simulink model "att_control_OneModule_V6"  (R2022a)
settings: Solver=ode15s  StartTime=0.0  StopTime=10  FixedStep=0.001  RelTol=1e-3
values from neighbouring files (symbols this model uses):
  act_lo = 0    [rotors_prg.m]
  act_up = 1000    [rotors_prg.m]
  des_alt = 1    [rotors_prg.m]
  des_p = 0    [rotors_prg.m]
  des_r = 0    [rotors_prg.m]
  des_y = 0    [rotors_prg.m]
  dragCoeffMov = 0    [rotors_prg.m]
  g = 9.81    [rotors_prg.m]
  KDx = 0.003*1    (= 0.003)    [rotors_prg.m]
  KDy = 0.003*1    (= 0.003)    [rotors_prg.m]
  KDz = 0.003*1    (= 0.003)    [rotors_prg.m]
  KIx = 0.2*1    (= 0.2)    [rotors_prg.m]
  KIy = 0.2*1    (= 0.2)    [rotors_prg.m]
  KIz = 0.2*1    (= 0.2)    [rotors_prg.m]
  KP1x = 6.5    [rotors_prg.m]
  KP1y = 6.5    [rotors_prg.m]
  KP1z = 2.8    [rotors_prg.m]
  KP2x = 0.15^1    (= 0.15)    [rotors_prg.m]
  KP2y = 0.15^1    (= 0.15)    [rotors_prg.m]
  KP2z = 0.15^1    (= 0.15)    [rotors_prg.m]
  mass = 16*mass1    (= 14.24)    [rotors_prg.m]
  Mv = inv(M)    [rotors_prg.m]
  rotorDir = rotorDirX    [rotors_prg.m]
  rotorPositions = rotorPositions16    [rotors_prg.m]
  rotorThrustMax = 5.3    [rotors_prg.m]
  rotorTimeConst = 0.005    [rotors_prg.m]
  rotorTorqueMax = 0.078    [rotors_prg.m]
  windVel = [0;0;0]    [rotors_prg.m]
undefined symbols (not defined in the file or in its folder): init
libraries: slpidlib x10, sharedtransform x3, simulink x2, aerolibutil x2, shared6dof x1, sharedutil x1
(part 1 of 2)
settings Model: Creator=MohShahab  LastModifiedBy=MohShahab
settings SolverCC: ZeroCrossAlgorithm=Adaptive
settings DebuggingCC: MaskedZcDiagnostic=none  IgnoredZcDiagnostic=none
settings SFSimCC: SimTargetLang=C++

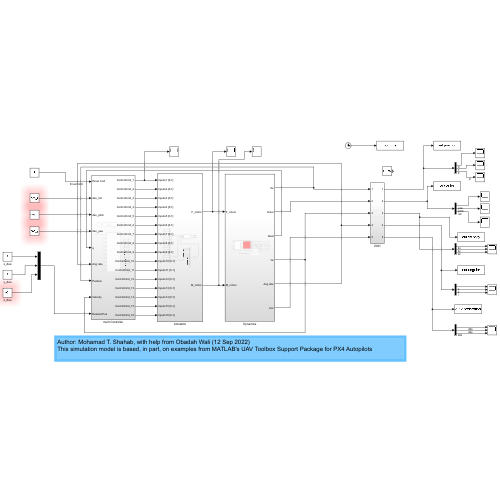
[thumbnail: Simulink's stored preview of the top-level diagram]
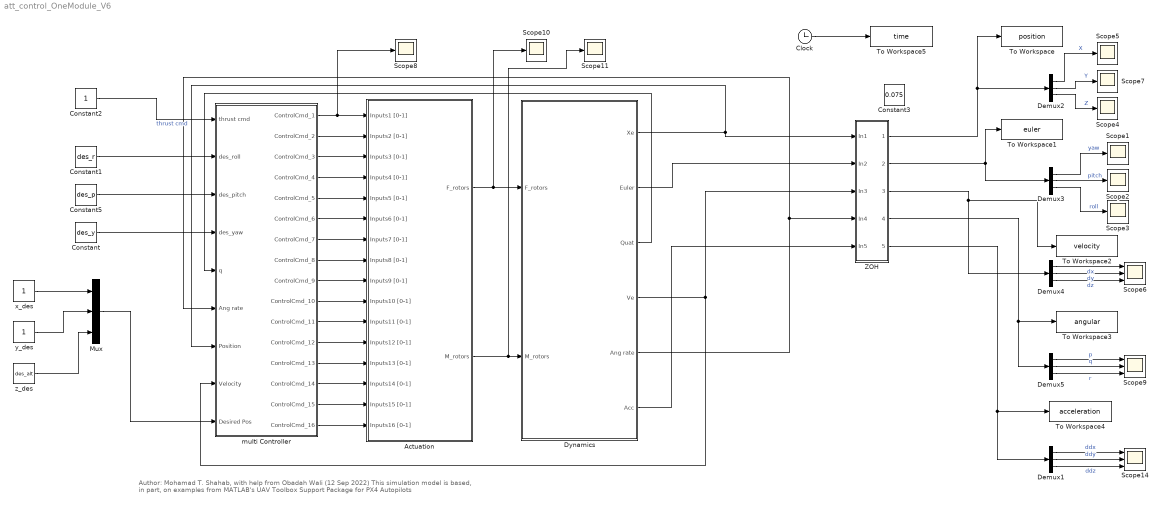
== system att_control_OneModule_V6 ==
  note: Author: Mohamad T. Shahab, with help from Obadah Wali (12 Sep 2022)
      | This simulation model is based, in part, on examples from MATLAB's UAV Toolbox Support Package for PX4 Autopilots
  Actuation : Subsystem
  Clock : Clock
  Constant : Constant  Value=des_y
  Constant1 : Constant  Value=des_r
  Constant2 : Constant
  Constant3 : Constant  Value=0.075
  Constant5 : Constant  Value=des_p
  Demux{1..5} (5 alike) : Demux  Outputs=3
  Dynamics : Subsystem
  Mux : Mux  Inputs=3
  Scope{1..5,7..8,10..11} (9 alike) : Scope
  Scope14 : Scope  NumInputPorts=3
  Scope6 : Scope  NumInputPorts=3
  Scope9 : Scope  NumInputPorts=3
  To Workspace : ToWorkspace  VariableName=position  SaveFormat=Timeseries  SampleTime=-1
  To Workspace1 : ToWorkspace  VariableName=euler  SaveFormat=Timeseries  SampleTime=-1
  To Workspace2 : ToWorkspace  VariableName=velocity  SaveFormat=Timeseries  SampleTime=-1
  To Workspace3 : ToWorkspace  VariableName=angular  SaveFormat=Timeseries  SampleTime=-1
  To Workspace4 : ToWorkspace  VariableName=acceleration  SaveFormat=Timeseries  SampleTime=-1
  To Workspace5 : ToWorkspace  VariableName=time  SaveFormat=Timeseries  SampleTime=-1
  ZOH : Subsystem
  multi Controller : Subsystem
  x_des : Constant
  y_des : Constant
  z_des : Constant  Value=des_alt
  wires:
  Demux5/3 -> Scope9/3  "r"
  Demux4/3 -> Scope6/3  "dz"
  Demux5/2 -> Scope9/2  "q"
  Demux4/1 -> Scope6/1  "dx"
  Demux5/1 -> Scope9/1  "p"
  Demux1/2 -> Scope14/2  "ddy"
  Demux1/1 -> Scope14/1  "ddx"
  Demux2/3 -> Scope4/1  "Z"
  Demux1/3 -> Scope14/3  "ddz"
  Demux4/2 -> Scope6/2  "dy"
  Dynamics/5(Ang rate) -> ZOH/4(In4), multi Controller/6(Ang rate)
  Constant2/1 -> multi Controller/1(thrust cmd)  "thrust cmd"
  Constant1/1 -> multi Controller/2(des_roll)
  Dynamics/3(Quat) -> multi Controller/5(q)
  Constant/1 -> multi Controller/4(des_yaw)
  Constant5/1 -> multi Controller/3(des_pitch)
  Dynamics/1(Xe) -> ZOH/1(In1), multi Controller/7(Position)
  Dynamics/2(Euler) -> ZOH/2(In2)
  Dynamics/4(Ve) -> multi Controller/8(Velocity), ZOH/3(In3)
  Dynamics/6(Acc) -> ZOH/5(In5)
  ZOH/1(Out1) -> Demux2/1, To Workspace/1
  ZOH/3(Out3) -> Demux4/1, To Workspace2/1
  ZOH/4(Out4) -> To Workspace3/1, Demux5/1
  ZOH/5(Out5) -> To Workspace4/1, Demux1/1
  Mux/1 -> multi Controller/9(Desired Pos)
  x_des/1 -> Mux/1
  y_des/1 -> Mux/2
  z_des/1 -> Mux/3
  Demux3/1 -> Scope1/1  "yaw"
  ZOH/2(Out2) -> To Workspace1/1, Demux3/1
  Demux3/2 -> Scope2/1  "pitch"
  multi Controller/1(ControlCmd_1) -> Scope8/1, Actuation/1(Inputs1 [0-1])
  Actuation/1(F_rotors) -> Scope10/1, Dynamics/1(F_rotors)
  Actuation/2(M_rotors) -> Scope11/1, Dynamics/2(M_rotors)
  multi Controller/2(ControlCmd_2) -> Actuation/2(Inputs2 [0-1])
  multi Controller/3(ControlCmd_3) -> Actuation/3(Inputs3 [0-1])
  multi Controller/4(ControlCmd_4) -> Actuation/4(Inputs4 [0-1])
  multi Controller/5(ControlCmd_5) -> Actuation/5(Inputs5 [0-1])
  multi Controller/6(ControlCmd_6) -> Actuation/6(Inputs6 [0-1])
  multi Controller/7(ControlCmd_7) -> Actuation/7(Inputs7 [0-1])
  multi Controller/8(ControlCmd_8) -> Actuation/8(Inputs8 [0-1])
  multi Controller/9(ControlCmd_9) -> Actuation/9(Inputs9 [0-1])
  multi Controller/10(ControlCmd_10) -> Actuation/10(Inputs10 [0-1])
  multi Controller/11(ControlCmd_11) -> Actuation/11(Inputs11 [0-1])
  multi Controller/12(ControlCmd_12) -> Actuation/12(Inputs12 [0-1])
  multi Controller/13(ControlCmd_13) -> Actuation/13(Inputs13 [0-1])
  multi Controller/14(ControlCmd_14) -> Actuation/14(Inputs14 [0-1])
  multi Controller/15(ControlCmd_15) -> Actuation/15(Inputs15 [0-1])
  multi Controller/16(ControlCmd_16) -> Actuation/16(Inputs16 [0-1])
  Demux2/1 -> Scope5/1  "X"
  Demux2/2 -> Scope7/1  "Y"
  Clock/1 -> To Workspace5/1
  Demux3/3 -> Scope3/1  "roll"

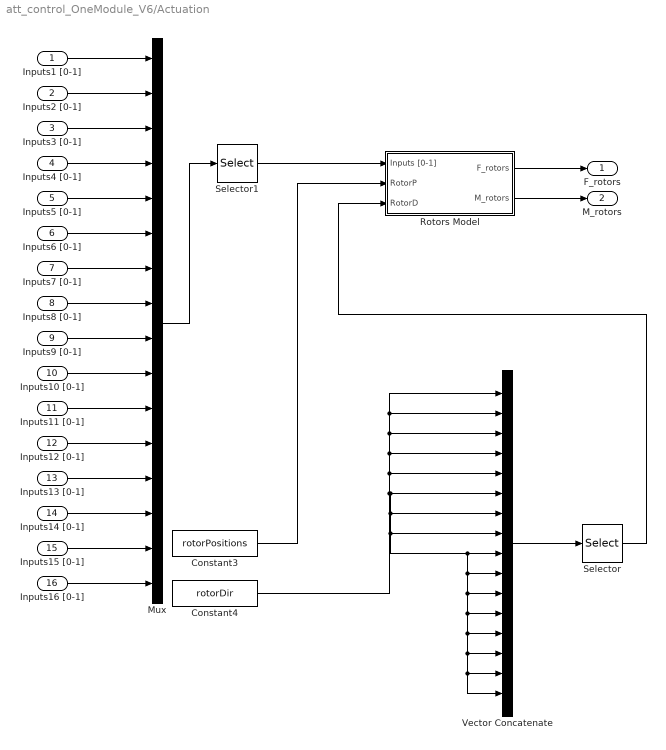
== system att_control_OneModule_V6/Actuation ==
  Inputs1 [0-1] : Inport
  Inputs2 [0-1] : Inport  Port=2
  Inputs3 [0-1] : Inport  Port=3
  Inputs4 [0-1] : Inport  Port=4
  Inputs5 [0-1] : Inport  Port=5
  Inputs6 [0-1] : Inport  Port=6
  Inputs7 [0-1] : Inport  Port=7
  Inputs8 [0-1] : Inport  Port=8
  Inputs9 [0-1] : Inport  Port=9
  Inputs10 [0-1] : Inport  Port=10
  Inputs11 [0-1] : Inport  Port=11
  Inputs12 [0-1] : Inport  Port=12
  Inputs13 [0-1] : Inport  Port=13
  Inputs14 [0-1] : Inport  Port=14
  Inputs15 [0-1] : Inport  Port=15
  Inputs16 [0-1] : Inport  Port=16
  Constant3 : Constant  Value=rotorPositions
  Constant4 : Constant  Value=rotorDir
  Mux : Mux  Inputs=16
  Rotors Model : Subsystem
  Selector : Selector  InputPortWidth=64  IndexOptions=Starting index (dialog)  Indices=1  OutputSizes=NumRotors
  Selector1 : Selector  InputPortWidth=64  IndexOptions=Starting index (dialog)  Indices=1  OutputSizes=NumRotors
  Vector Concatenate : Concatenate  NumInputs=16
  F_rotors : Outport
  M_rotors : Outport  Port=2
  wires:
  Rotors Model/2(M_rotors) -> M_rotors/1
  Rotors Model/1(F_rotors) -> F_rotors/1
  Inputs3 [0-1]/1 -> Mux/3
  Inputs4 [0-1]/1 -> Mux/4
  Constant3/1 -> Rotors Model/2(RotorP)
  Inputs7 [0-1]/1 -> Mux/7
  Inputs8 [0-1]/1 -> Mux/8
  Inputs6 [0-1]/1 -> Mux/6
  Inputs5 [0-1]/1 -> Mux/5
  Inputs11 [0-1]/1 -> Mux/11
  Inputs12 [0-1]/1 -> Mux/12
  Inputs10 [0-1]/1 -> Mux/10
  Inputs9 [0-1]/1 -> Mux/9
  Inputs15 [0-1]/1 -> Mux/15
  Inputs16 [0-1]/1 -> Mux/16
  Inputs14 [0-1]/1 -> Mux/14
  Inputs13 [0-1]/1 -> Mux/13
  Constant4/1 -> Vector Concatenate/2, Vector Concatenate/1, Vector Concatenate/3, Vector Concatenate/4, Vector Concatenate/5, Vector Concatenate/16, Vector Concatenate/15, Vector Concatenate/14, Vector Concatenate/13, Vector Concatenate/12, Vector Concatenate/11, Vector Concatenate/10, Vector Concatenate/9, Vector Concatenate/8, Vector Concatenate/7, Vector Concatenate/6
  Vector Concatenate/1 -> Selector/1
  Selector/1 -> Rotors Model/3(RotorD)
  Mux/1 -> Selector1/1
  Selector1/1 -> Rotors Model/1(Inputs [0-1])
  Inputs2 [0-1]/1 -> Mux/2
  Inputs1 [0-1]/1 -> Mux/1

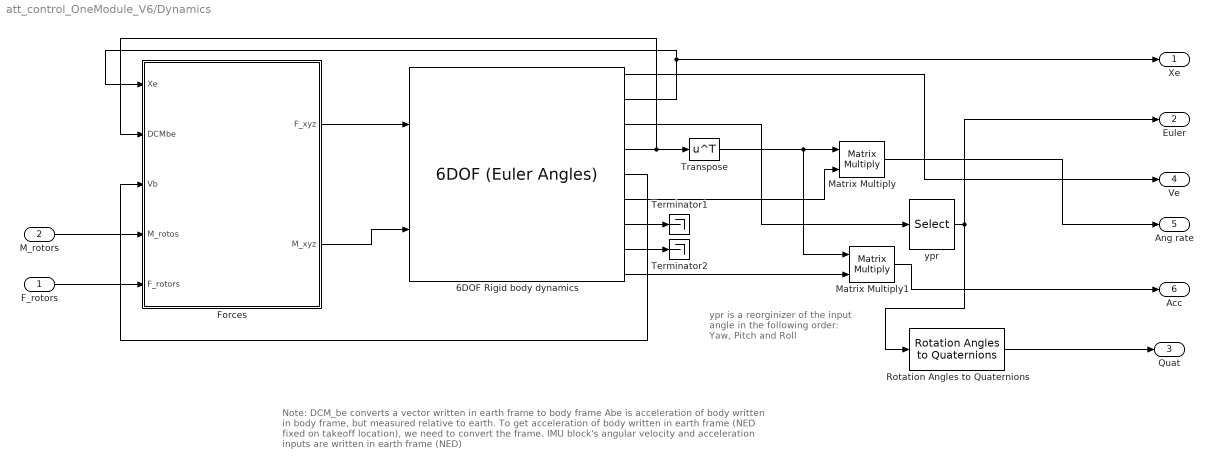
== system att_control_OneModule_V6/Dynamics ==
  note: Note:
      | DCM_be converts a vector written in earth frame to body frame
      | Abe is acceleration of body written in body frame, but measured relative to earth.
      | To get acceleration of body written in earth frame (NED fixed on takeoff location), we need to convert the frame.
      | IMU block's angular velocity and acceleration inputs are written in earth frame (NED)
  note: ypr is a reorginizer of the input angle in the following order: Yaw, Pitch and Roll
  F_rotors : Inport
  M_rotors : Inport  Port=2
  "6DOF Rigid body dynamics " : shared6dof/6DOF (Euler Angles)  units=Metric (MKS)  mtype=Fixed  rep=Quaternion  xme_0=init.posNED  Vm_0=init.vb  eul_0=init.euler  pm_0=init.angRates  mass_0=mass  mass_e=0.5  mass_f=2.0  inertia=inertia  inertia_e=eye(3)  inertia_f=2*eye(3)  k_quat=1  vre_flag=on  abi_flag=on  aMode=aMode  xme_statename=''  Vm_statename=''  eul_statename=''  quat_statename=''  pm_statename=''  mass_statename=''
      settings: SourceProductBaseCode=AE,PW,DR,MT,VE
  Forces : Subsystem
  Matrix Multiply : Product  Multiplication=Matrix(*)
  Matrix Multiply1 : Product  Multiplication=Matrix(*)
  Rotation Angles to Quaternions : sharedtransform/Rotation Angles to Quaternions  rotationOrder=ZYX  aMode=aMode
      settings: SourceProductBaseCode=AE,PW,DR,MT,VE
  Terminator1 : Terminator
  Terminator2 : Terminator
  Transpose : Math  Operator=transpose
  ypr : Selector  InputPortWidth=3  IndexOptions=Index vector (dialog)  Indices=[3 2 1]  OutputSizes=1
  Xe : Outport
  Euler : Outport  Port=2
  Quat : Outport  Port=3
  Ve : Outport  Port=4
  Ang rate : Outport  Port=5
  Acc : Outport  Port=6
  wires:
  Transpose/1 -> Matrix Multiply1/1, Matrix Multiply/1
  ypr/1 -> Euler/1, Rotation Angles to Quaternions/1
  "6DOF Rigid body dynamics "/4 -> Forces/2(DCMbe), Transpose/1
  "6DOF Rigid body dynamics "/2 -> Xe/1, Forces/1(Xe)
  "6DOF Rigid body dynamics "/3 -> ypr/1
  "6DOF Rigid body dynamics "/1 -> Ve/1
  "6DOF Rigid body dynamics "/8 -> Terminator2/1
  "6DOF Rigid body dynamics "/6 -> Matrix Multiply/2
  "6DOF Rigid body dynamics "/9 -> Matrix Multiply1/2
  "6DOF Rigid body dynamics "/7 -> Terminator1/1
  "6DOF Rigid body dynamics "/5 -> Forces/3(Vb)
  Forces/1(F_xyz) -> "6DOF Rigid body dynamics "/1
  Forces/2(M_xyz) -> "6DOF Rigid body dynamics "/2
  Matrix Multiply/1 -> Ang rate/1
  Matrix Multiply1/1 -> Acc/1
  M_rotors/1 -> Forces/4(M_rotos)
  Rotation Angles to Quaternions/1 -> Quat/1
  F_rotors/1 -> Forces/5(F_rotors)

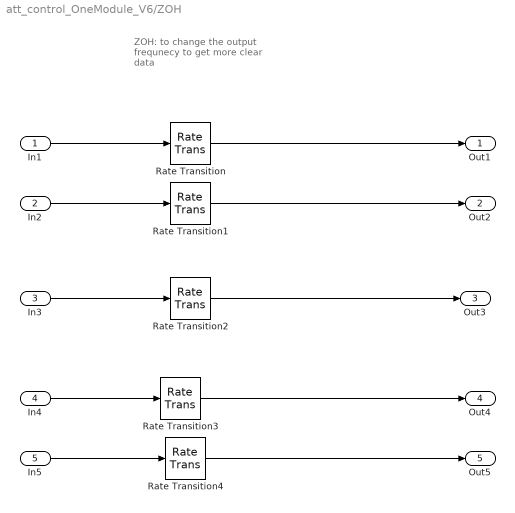
== system att_control_OneModule_V6/ZOH ==
  note: ZOH: to change the output frequnecy to get more clear data
  In1 : Inport
  In2 : Inport  Port=2
  In3 : Inport  Port=3
  In4 : Inport  Port=4
  In5 : Inport  Port=5
  Rate Transition{,1..4} (5 alike) : RateTransition  OutPortSampleTime=SampleTime
  Out1 : Outport
  Out2 : Outport  Port=2
  Out3 : Outport  Port=3
  Out4 : Outport  Port=4
  Out5 : Outport  Port=5
  wires:
  In4/1 -> Rate Transition3/1
  Rate Transition2/1 -> Out3/1
  Rate Transition/1 -> Out1/1
  Rate Transition4/1 -> Out5/1
  Rate Transition3/1 -> Out4/1
  Rate Transition1/1 -> Out2/1
  In1/1 -> Rate Transition/1
  In5/1 -> Rate Transition4/1
  In2/1 -> Rate Transition1/1
  In3/1 -> Rate Transition2/1

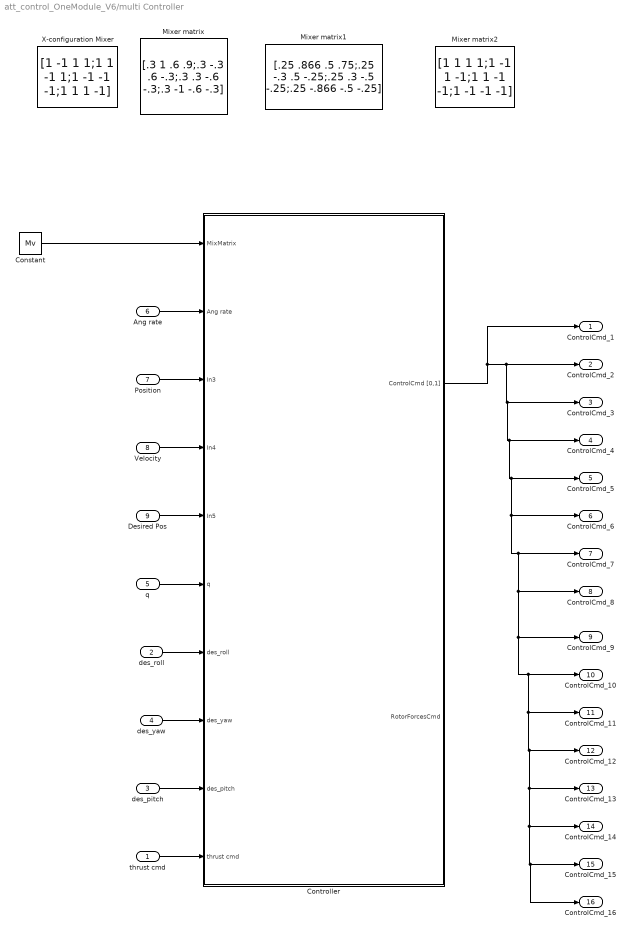
== system att_control_OneModule_V6/multi Controller ==
  thrust cmd : Inport
  des_roll : Inport  Port=2
  des_pitch : Inport  Port=3
  des_yaw : Inport  Port=4
  q : Inport  Port=5
  Ang rate : Inport  Port=6
  Position : Inport  Port=7
  Velocity : Inport  Port=8
  Desired Pos : Inport  Port=9
  Constant : Constant  Value=Mv
  Controller : Subsystem
  Mixer matrix : Constant  Value=[.3 1 .6 .9;.3 -.3 .6 -.3;.3 .3 -.6 -.3;.3 -1 -.6 -.3]  OutDataTypeStr=Inherit: Inherit via back propagation  SampleTime=-1
  Mixer matrix1 : Constant  Value=[.25 .866 .5 .75;.25 -.3 .5 -.25;.25 .3 -.5 -.25;.25 -.866 -.5 -.25]  OutDataTypeStr=Inherit: Inherit via back propagation  SampleTime=-1
  Mixer matrix2 : Constant  Value=[1 1 1 1;1 -1 1 -1;1 1 -1 -1;1 -1 -1 -1]  OutDataTypeStr=Inherit: Inherit via back propagation  SampleTime=-1
  "X-configuration Mixer " : Constant  Value=[1 -1 1 1;1 1 -1 1;1 -1 -1 -1;1 1 1 -1]  OutDataTypeStr=Inherit: Inherit via back propagation  SampleTime=-1
  ControlCmd_1 : Outport
  ControlCmd_2 : Outport  Port=2
  ControlCmd_3 : Outport  Port=3
  ControlCmd_4 : Outport  Port=4
  ControlCmd_5 : Outport  Port=5
  ControlCmd_6 : Outport  Port=6
  ControlCmd_7 : Outport  Port=7
  ControlCmd_8 : Outport  Port=8
  ControlCmd_9 : Outport  Port=9
  ControlCmd_10 : Outport  Port=10
  ControlCmd_11 : Outport  Port=11
  ControlCmd_12 : Outport  Port=12
  ControlCmd_13 : Outport  Port=13
  ControlCmd_14 : Outport  Port=14
  ControlCmd_15 : Outport  Port=15
  ControlCmd_16 : Outport  Port=16
  wires:
  Ang rate/1 -> Controller/2(Ang rate)
  Position/1 -> Controller/3(In3)
  Velocity/1 -> Controller/4(In4)
  Desired Pos/1 -> Controller/5(In5)
  q/1 -> Controller/6(q)
  des_roll/1 -> Controller/7(des_roll)
  des_yaw/1 -> Controller/8(des_yaw)
  des_pitch/1 -> Controller/9(des_pitch)
  Controller/1(ControlCmd [0,1]) -> ControlCmd_1/1, ControlCmd_16/1, ControlCmd_15/1, ControlCmd_14/1, ControlCmd_13/1, ControlCmd_12/1, ControlCmd_11/1, ControlCmd_10/1, ControlCmd_9/1, ControlCmd_8/1, ControlCmd_7/1, ControlCmd_6/1, ControlCmd_5/1, ControlCmd_4/1, ControlCmd_3/1, ControlCmd_2/1
  Constant/1 -> Controller/1(MixMatrix)
  thrust cmd/1 -> Controller/10(thrust cmd)

== system att_control_OneModule_V6/Actuation/Rotors Model ==
  Inputs [0-1] : Inport
  RotorP : Inport  Port=2
  RotorD : Inport  Port=3
  MATLAB Function : MATLAB Function  TreatAsAtomicUnit=on
  Thrust model : Subsystem
  Torque model : Subsystem
  F_rotors : Outport
  M_rotors : Outport  Port=2
  wires:
  Inputs [0-1]/1 -> Torque model/1(In1), Thrust model/1(In1)
  MATLAB Function/1(netF) -> F_rotors/1
  MATLAB Function/2(netM) -> M_rotors/1
  RotorP/1 -> MATLAB Function/3(rotorPositions)
  RotorD/1 -> MATLAB Function/4(rotorDir)
  Thrust model/1(thrustEachRotor) -> MATLAB Function/1(thrustEachRotor)
  Torque model/1(tauEachRotor) -> MATLAB Function/2(tauEachRotor)

== system att_control_OneModule_V6/Dynamics/Forces ==
  Xe : Inport
  DCMbe : Inport  Port=2
  Vb : Inport  Port=3
  M_rotos : Inport  Port=4
  F_rotors : Inport  Port=5
  Force and Moment Calculation : Subsystem
  F_xyz : Outport
  M_xyz : Outport  Port=2
  wires:
  DCMbe/1 -> Force and Moment Calculation/1(DCMbe)
  Force and Moment Calculation/1(F_xyz) -> F_xyz/1
  Vb/1 -> Force and Moment Calculation/2(Vb)
  Force and Moment Calculation/2(M_xyz) -> M_xyz/1
  Xe/1 -> Force and Moment Calculation/3(Xe)
  F_rotors/1 -> Force and Moment Calculation/4(F_total)
  M_rotos/1 -> Force and Moment Calculation/5(M_total)

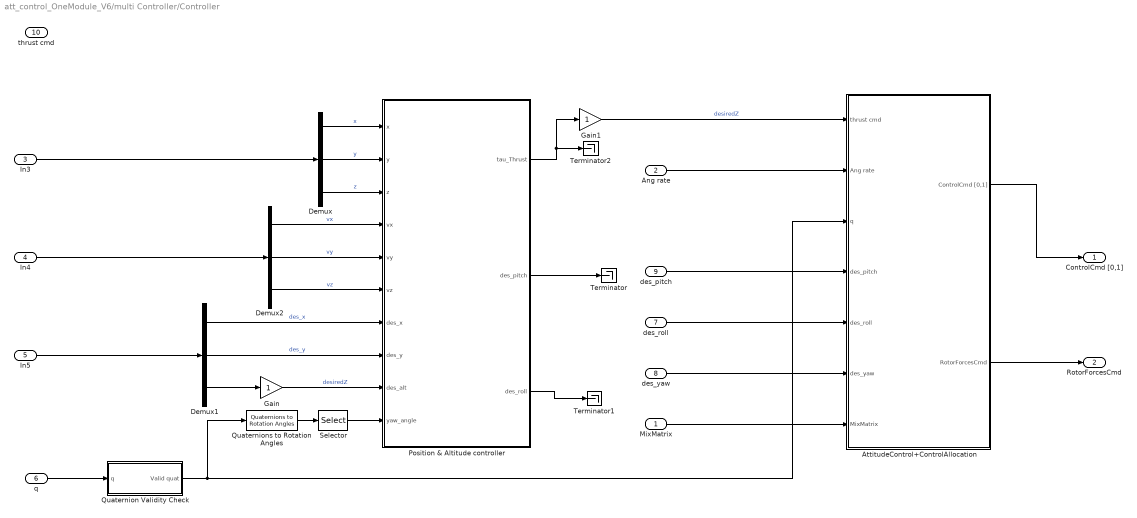
== system att_control_OneModule_V6/multi Controller/Controller ==
  MixMatrix : Inport
  Ang rate : Inport  Port=2
  In3 : Inport  Port=3
  In4 : Inport  Port=4
  In5 : Inport  Port=5
  q : Inport  Port=6
  des_roll : Inport  Port=7
  des_yaw : Inport  Port=8
  des_pitch : Inport  Port=9
  thrust cmd : Inport  Port=10
  AttitudeControl+ControlAllocation : Subsystem
  Demux : Demux  Outputs=3
  Demux1 : Demux  Outputs=3
  Demux2 : Demux  Outputs=3
  Gain : Gain
  Gain1 : Gain
  Position & Altitude controller : Subsystem
  Quaternion Validity Check : Subsystem
  Quaternions to Rotation Angles : sharedtransform/Quaternions to Rotation Angles  rotationOrder=ZYX  aMode=aMode
      settings: SourceProductBaseCode=AE,PW,DR,MT,VE
  Selector : Selector  InputPortWidth=3  IndexOptions=Index vector (dialog)  Indices=[1]  OutputSizes=1
  Terminator : Terminator
  Terminator1 : Terminator
  Terminator2 : Terminator
  ControlCmd [0,1] : Outport
  RotorForcesCmd : Outport  Port=2
  wires:
  Demux/2 -> Position & Altitude controller/2(y)  "y"
  Position & Altitude controller/2(des_pitch) -> Terminator/1
  Demux1/3 -> Gain/1
  Position & Altitude controller/1(tau_Thrust) -> Gain1/1, Terminator2/1
  Position & Altitude controller/3(des_roll) -> Terminator1/1
  Gain/1 -> Position & Altitude controller/9(des_alt)  "desiredZ"
  Quaternions to Rotation Angles/1 -> Selector/1
  Quaternion Validity Check/1(Valid quat) -> Quaternions to Rotation Angles/1, AttitudeControl+ControlAllocation/3(q)
  Demux1/2 -> Position & Altitude controller/8(des_y)  "des_y"
  In5/1 -> Demux1/1
  Selector/1 -> Position & Altitude controller/10(yaw_angle)
  Demux/3 -> Position & Altitude controller/3(z)  "z"
  In3/1 -> Demux/1
  Demux1/1 -> Position & Altitude controller/7(des_x)  "des_x"
  Demux2/2 -> Position & Altitude controller/5(vy)  "vy"
  Demux2/1 -> Position & Altitude controller/4(vx)  "vx"
  Demux2/3 -> Position & Altitude controller/6(vz)  "vz"
  Demux/1 -> Position & Altitude controller/1(x)  "x"
  MixMatrix/1 -> AttitudeControl+ControlAllocation/7(MixMatrix)
  q/1 -> Quaternion Validity Check/1(q)
  des_yaw/1 -> AttitudeControl+ControlAllocation/6(des_yaw)
  Ang rate/1 -> AttitudeControl+ControlAllocation/2(Ang rate)
  In4/1 -> Demux2/1
  AttitudeControl+ControlAllocation/2(RotorForcesCmd) -> RotorForcesCmd/1
  AttitudeControl+ControlAllocation/1(ControlCmd [0,1]) -> ControlCmd [0,1]/1
  Gain1/1 -> AttitudeControl+ControlAllocation/1(thrust cmd)  "desiredZ"
  des_pitch/1 -> AttitudeControl+ControlAllocation/4(des_pitch)
  des_roll/1 -> AttitudeControl+ControlAllocation/5(des_roll)

== system att_control_OneModule_V6/Actuation/Rotors Model/Thrust model ==
  In1 : Inport
  Demux : Demux
  Mux : Mux
  Transfer Fcn{,2..4} (4 alike) : TransferFcn  Numerator=[rotorThrustMax]  Denominator=[rotorTimeConst 1]
  thrustEachRotor : Outport
  wires:
  Transfer Fcn3/1 -> Mux/2
  Demux/1 -> Transfer Fcn4/1
  Transfer Fcn2/1 -> Mux/3
  Demux/3 -> Transfer Fcn2/1
  Mux/1 -> thrustEachRotor/1
  Transfer Fcn4/1 -> Mux/1
  Demux/4 -> Transfer Fcn/1
  Demux/2 -> Transfer Fcn3/1
  Transfer Fcn/1 -> Mux/4
  In1/1 -> Demux/1

== system att_control_OneModule_V6/Actuation/Rotors Model/Torque model ==
  In1 : Inport
  Demux : Demux
  Mux : Mux
  Transfer Fcn{1..4} (4 alike) : TransferFcn  Numerator=[rotorTorqueMax]  Denominator=[rotorTimeConst 1]
  tauEachRotor : Outport
  wires:
  Transfer Fcn4/1 -> Mux/4
  Demux/1 -> Transfer Fcn1/1
  Transfer Fcn3/1 -> Mux/3
  Transfer Fcn2/1 -> Mux/2
  Demux/2 -> Transfer Fcn2/1
  Demux/4 -> Transfer Fcn4/1
  Demux/3 -> Transfer Fcn3/1
  Mux/1 -> tauEachRotor/1
  Transfer Fcn1/1 -> Mux/1
  In1/1 -> Demux/1

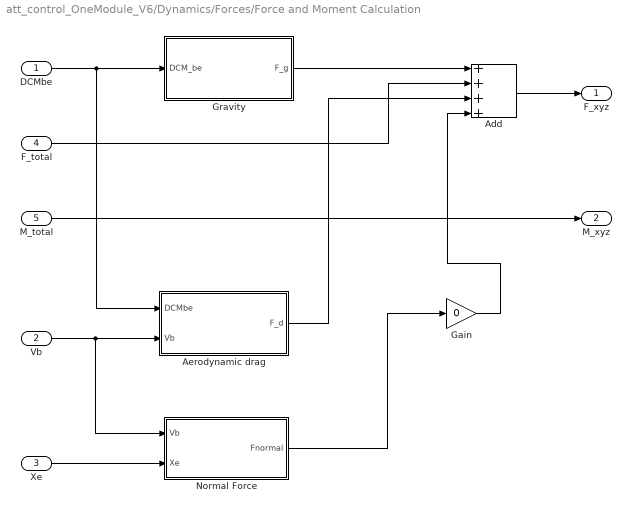
== system att_control_OneModule_V6/Dynamics/Forces/Force and Moment Calculation ==
  DCMbe : Inport
  Vb : Inport  Port=2
  Xe : Inport  Port=3
  F_total : Inport  Port=4
  M_total : Inport  Port=5
  Add : Sum  Inputs=++++
  Aerodynamic drag : Subsystem
  Gain : Gain  Gain=0
  Gravity : Subsystem
  Normal Force : Subsystem
  F_xyz : Outport
  M_xyz : Outport  Port=2
  wires:
  DCMbe/1 -> Aerodynamic drag/1(DCMbe), Gravity/1(DCM_be)
  Gravity/1(F_g) -> Add/1
  Add/1 -> F_xyz/1
  Vb/1 -> Aerodynamic drag/2(Vb), Normal Force/1(Vb)
  Aerodynamic drag/1(F_d) -> Add/3
  Xe/1 -> Normal Force/2(Xe)
  Normal Force/1(Fnormal) -> Gain/1
  Gain/1 -> Add/4
  M_total/1 -> M_xyz/1
  F_total/1 -> Add/2

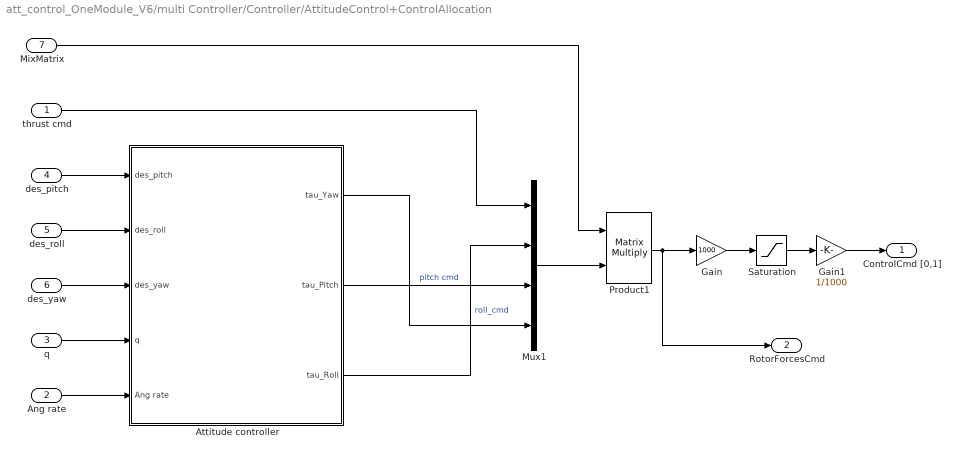
== system att_control_OneModule_V6/multi Controller/Controller/AttitudeControl+ControlAllocation ==
  thrust cmd : Inport
  Ang rate : Inport  Port=2
  q : Inport  Port=3
  des_pitch : Inport  Port=4
  des_roll : Inport  Port=5
  des_yaw : Inport  Port=6
  MixMatrix : Inport  Port=7
  Attitude controller : Subsystem
  Gain : Gain  Gain=1000
  Gain1 : Gain  Gain=1/1000
  Mux1 : Mux
  Product1 : Product  Multiplication=Matrix(*)  RndMeth=Zero
  Saturation : Saturate  UpperLimit=act_up  LowerLimit=act_lo  LinearizeAsGain=off  ZeroCross=off
      settings: LockScale=on
  ControlCmd [0,1] : Outport
  RotorForcesCmd : Outport  Port=2
  wires:
  des_pitch/1 -> Attitude controller/1(des_pitch)
  q/1 -> Attitude controller/4(q)
  Ang rate/1 -> Attitude controller/5(Ang rate)
  thrust cmd/1 -> Mux1/1
  des_roll/1 -> Attitude controller/2(des_roll)
  Mux1/1 -> Product1/2
  des_yaw/1 -> Attitude controller/3(des_yaw)
  MixMatrix/1 -> Product1/1
  Attitude controller/1(tau_Yaw) -> Mux1/4
  Attitude controller/2(tau_Pitch) -> Mux1/3  "pitch cmd"
  Attitude controller/3(tau_Roll) -> Mux1/2  "roll_cmd"
  Product1/1 -> RotorForcesCmd/1, Gain/1
  Saturation/1 -> Gain1/1
  Gain/1 -> Saturation/1
  Gain1/1 -> ControlCmd [0,1]/1

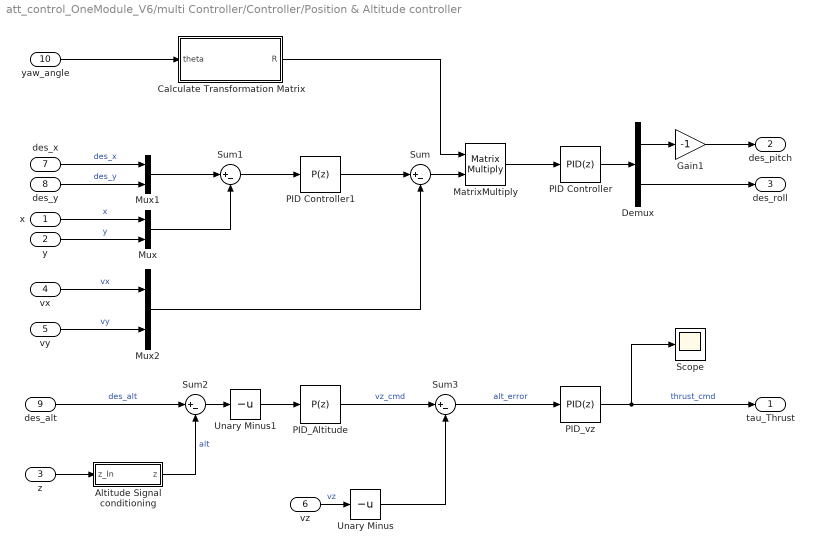
== system att_control_OneModule_V6/multi Controller/Controller/Position & Altitude controller ==
  x : Inport
  y : Inport  Port=2
  z : Inport  Port=3
  vx : Inport  Port=4
  vy : Inport  Port=5
  vz : Inport  Port=6
  des_x : Inport  Port=7
  des_y : Inport  Port=8
  des_alt : Inport  Port=9
  yaw_angle : Inport  Port=10
  Altitude Signal conditioning : Subsystem
  Calculate Transformation Matrix : Subsystem
  Demux : Demux  Outputs=2
  Gain1 : Gain  Gain=-1
  MatrixMultiply : Product  Multiplication=Matrix(*)
  Mux : Mux  Inputs=2
  Mux1 : Mux  Inputs=2
  Mux2 : Mux  Inputs=2
  PID Controller : slpidlib/PID Controller  Controller=PID  Form=Parallel  TimeDomain=Discrete-time  UseExternalTs=off  SampleTime=-1  IntegratorMethod=Forward Euler  FilterMethod=Forward Euler  ControllerParametersSource=internal  P=1.8  I=0.4  UseKiTs=off  D=0.2  N=20  UseFilter=on  TunerSelectOption=Transfer Function Based (PID Tuner App)  InitialConditionSource=internal  InitialConditionForIntegrator=0  InitialConditionForFilter=0  DifferentiatorICPrevScaledInput=0  ExternalReset=none  TrackingMode=off  Kt=1  LimitOutput=on  SatLimitsSource=internal  UpperSaturationLimit=20*pi/180  LowerSaturationLimit=-20*pi/180  LinearizeAsGain=on  AntiWindupMode=clamping  Kb=1  POutMin=[]  POutMax=[]  IOutMin=[]  IOutMax=[]  DOutMin=[]  DOutMax=[]  NOutMin=[]  NOutMax=[]  SumOutMin=[]  SumOutMax=[]  SaturationOutMin=[]  SaturationOutMax=[]  PParamMin=[]  PParamMax=[]  IParamMin=[]  IParamMax=[]  DParamMin=[]  DParamMax=[]  NParamMin=[]  NParamMax=[]  KbParamMin=[]  KbParamMax=[]  KtParamMin=[]  KtParamMax=[]  KbOutMin=[]  KbOutMax=[]  KtOutMin=[]  KtOutMax=[]  IntegratorOutMin=[]  IntegratorOutMax=[]  FilterOutMin=[]  FilterOutMax=[]  SumI1OutMin=[]  SumI1OutMax=[]  SumI2OutMin=[]  SumI2OutMax=[]  SumI3OutMin=[]  SumI3OutMax=[]  SumI4OutMin=[]  SumI4OutMax=[]  SumDOutMin=[]  SumDOutMax=[]  DifferentiatorOutMin=[]  DifferentiatorOutMax=[]  FilterDiffOutCoefMin=[]  FilterDiffOutCoefMax=[]  ReciprocalOutMin=[]  ReciprocalOutMax=[]  SumDenOutMin=[]  SumDenOutMax=[]  SumNumOutMin=[]  SumNumOutMax=[]  DivideOutMin=[]  DivideOutMax=[]  UdiffTsProdOutMin=[]  UdiffTsProdOutMax=[]  NTsProdOutMin=[]  NTsProdOutMax=[]  UintegralTsProdOutMin=[]  UintegralTsProdOutMax=[]  UngainTsProdOutMin=[]  UngainTsProdOutMax=[]  IntegratorContinuousStateAttributes=''  IntegratorStateMustResolveToSignalObject=off  IntegratorRTWStateStorageClass=Auto  FilterContinuousStateAttributes=''  FilterStateMustResolveToSignalObject=off  FilterRTWStateStorageClass=Auto  ParallelPVariant=InternalParameters  IdealPVariant=Disabled  IVariant=InternalParameters  DVariant=InternalParameters  IntegratorVariant=Discrete  SatVariant=Enabled  AWVariant=DiscClampingParallel  PCopyVariant=Disabled  TRVariant=Disabled  FdbkBlocksVariant=Forward  IdealPFdbkVariant=Disabled  SatFdbkVariant=Disabled  DerivativeFilterVariant=ForwardEulerFilter  NVariant=InternalParameters  NCopyVariant=Disabled  FilterICVariant=InternalICsFilter  IntegratorICVariant=InternalICs  ExternalResetVariant=Disabled  TRSumVariant=Passthrough  SumFdbkVariant=Disabled  SumVariant=Sum_PID  TsampFilterVariant=InternalTs  TsampNgainVariant=Passthrough  TsampIntegralVariant=Passthrough  ExternalSaturationOutDataTypeStr=Inherit: Same as second input  aMode=0
  PID Controller1 : slpidlib/PID Controller  Controller=P  Form=Parallel  TimeDomain=Discrete-time  UseExternalTs=off  SampleTime=-1  IntegratorMethod=Forward Euler  FilterMethod=Forward Euler  ControllerParametersSource=internal  P=0.95  I=0  UseKiTs=off  D=0  N=20  UseFilter=on  TunerSelectOption=Transfer Function Based (PID Tuner App)  InitialConditionSource=internal  InitialConditionForIntegrator=0  InitialConditionForFilter=0  DifferentiatorICPrevScaledInput=0  ExternalReset=none  TrackingMode=off  Kt=1  LimitOutput=on  SatLimitsSource=internal  UpperSaturationLimit=12  LowerSaturationLimit=-12  LinearizeAsGain=on  AntiWindupMode=clamping  Kb=1  POutMin=[]  POutMax=[]  IOutMin=[]  IOutMax=[]  DOutMin=[]  DOutMax=[]  NOutMin=[]  NOutMax=[]  SumOutMin=[]  SumOutMax=[]  SaturationOutMin=[]  SaturationOutMax=[]  PParamMin=[]  PParamMax=[]  IParamMin=[]  IParamMax=[]  DParamMin=[]  DParamMax=[]  NParamMin=[]  NParamMax=[]  KbParamMin=[]  KbParamMax=[]  KtParamMin=[]  KtParamMax=[]  KbOutMin=[]  KbOutMax=[]  KtOutMin=[]  KtOutMax=[]  IntegratorOutMin=[]  IntegratorOutMax=[]  FilterOutMin=[]  FilterOutMax=[]  SumI1OutMin=[]  SumI1OutMax=[]  SumI2OutMin=[]  SumI2OutMax=[]  SumI3OutMin=[]  SumI3OutMax=[]  SumI4OutMin=[]  SumI4OutMax=[]  SumDOutMin=[]  SumDOutMax=[]  DifferentiatorOutMin=[]  DifferentiatorOutMax=[]  FilterDiffOutCoefMin=[]  FilterDiffOutCoefMax=[]  ReciprocalOutMin=[]  ReciprocalOutMax=[]  SumDenOutMin=[]  SumDenOutMax=[]  SumNumOutMin=[]  SumNumOutMax=[]  DivideOutMin=[]  DivideOutMax=[]  UdiffTsProdOutMin=[]  UdiffTsProdOutMax=[]  NTsProdOutMin=[]  NTsProdOutMax=[]  UintegralTsProdOutMin=[]  UintegralTsProdOutMax=[]  UngainTsProdOutMin=[]  UngainTsProdOutMax=[]  IntegratorContinuousStateAttributes=''  IntegratorStateMustResolveToSignalObject=off  IntegratorRTWStateStorageClass=Auto  FilterContinuousStateAttributes=''  FilterStateMustResolveToSignalObject=off  FilterRTWStateStorageClass=Auto  ParallelPVariant=InternalParameters  IdealPVariant=Disabled  IVariant=Disabled  DVariant=Disabled  IntegratorVariant=Disabled  SatVariant=Enabled  AWVariant=Disabled  PCopyVariant=Disabled  TRVariant=Disabled  FdbkBlocksVariant=Forward  IdealPFdbkVariant=Disabled  SatFdbkVariant=Disabled  DerivativeFilterVariant=Disabled  NVariant=Disabled  NCopyVariant=Disabled_SignalSpec  FilterICVariant=Disabled  IntegratorICVariant=Disabled  ExternalResetVariant=Disabled  TRSumVariant=Passthrough  SumFdbkVariant=Disabled  SumVariant=Passthrough_P  TsampFilterVariant=InternalTs  TsampNgainVariant=Passthrough  TsampIntegralVariant=Disabled_SignalSpec  ExternalSaturationOutDataTypeStr=Inherit: Same as second input  aMode=0
  PID_Altitude : slpidlib/PID Controller  Controller=P  Form=Parallel  TimeDomain=Discrete-time  UseExternalTs=off  SampleTime=-1  IntegratorMethod=Backward Euler  FilterMethod=Forward Euler  ControllerParametersSource=internal  P=1.0*1  I=0.01*1  UseKiTs=off  D=0.01*1  N=10  UseFilter=on  TunerSelectOption=Transfer Function Based (PID Tuner App)  InitialConditionSource=internal  InitialConditionForIntegrator=0  InitialConditionForFilter=0  DifferentiatorICPrevScaledInput=0  ExternalReset=none  TrackingMode=off  Kt=1  LimitOutput=on  SatLimitsSource=internal  UpperSaturationLimit=2  LowerSaturationLimit=-2  LinearizeAsGain=on  AntiWindupMode=clamping  Kb=1  POutMin=[]  POutMax=[]  IOutMin=[]  IOutMax=[]  DOutMin=[]  DOutMax=[]  NOutMin=[]  NOutMax=[]  SumOutMin=[]  SumOutMax=[]  SaturationOutMin=[]  SaturationOutMax=[]  PParamMin=[]  PParamMax=[]  IParamMin=[]  IParamMax=[]  DParamMin=[]  DParamMax=[]  NParamMin=[]  NParamMax=[]  KbParamMin=[]  KbParamMax=[]  KtParamMin=[]  KtParamMax=[]  KbOutMin=[]  KbOutMax=[]  KtOutMin=[]  KtOutMax=[]  IntegratorOutMin=[]  IntegratorOutMax=[]  FilterOutMin=[]  FilterOutMax=[]  SumI1OutMin=[]  SumI1OutMax=[]  SumI2OutMin=[]  SumI2OutMax=[]  SumI3OutMin=[]  SumI3OutMax=[]  SumI4OutMin=[]  SumI4OutMax=[]  SumDOutMin=[]  SumDOutMax=[]  DifferentiatorOutMin=[]  DifferentiatorOutMax=[]  FilterDiffOutCoefMin=[]  FilterDiffOutCoefMax=[]  ReciprocalOutMin=[]  ReciprocalOutMax=[]  SumDenOutMin=[]  SumDenOutMax=[]  SumNumOutMin=[]  SumNumOutMax=[]  DivideOutMin=[]  DivideOutMax=[]  UdiffTsProdOutMin=[]  UdiffTsProdOutMax=[]  NTsProdOutMin=[]  NTsProdOutMax=[]  UintegralTsProdOutMin=[]  UintegralTsProdOutMax=[]  UngainTsProdOutMin=[]  UngainTsProdOutMax=[]  IntegratorContinuousStateAttributes=''  IntegratorStateMustResolveToSignalObject=off  IntegratorRTWStateStorageClass=Auto  FilterContinuousStateAttributes=''  FilterStateMustResolveToSignalObject=off  FilterRTWStateStorageClass=Auto  ParallelPVariant=InternalParameters  IdealPVariant=Disabled  IVariant=Disabled  DVariant=Disabled  IntegratorVariant=Disabled  SatVariant=Enabled  AWVariant=Disabled  PCopyVariant=Disabled  TRVariant=Disabled  FdbkBlocksVariant=Forward  IdealPFdbkVariant=Disabled  SatFdbkVariant=Disabled  DerivativeFilterVariant=Disabled  NVariant=Disabled  NCopyVariant=Disabled_SignalSpec  FilterICVariant=Disabled  IntegratorICVariant=Disabled  ExternalResetVariant=Disabled  TRSumVariant=Passthrough  SumFdbkVariant=Disabled  SumVariant=Passthrough_P  TsampFilterVariant=InternalTs  TsampNgainVariant=Passthrough  TsampIntegralVariant=Disabled_SignalSpec  ExternalSaturationOutDataTypeStr=Inherit: Same as second input  aMode=0
  PID_vz : slpidlib/PID Controller  Controller=PID  Form=Parallel  TimeDomain=Discrete-time  UseExternalTs=off  SampleTime=-1  IntegratorMethod=Backward Euler  FilterMethod=Forward Euler  ControllerParametersSource=internal  P=4  I=2  UseKiTs=off  D=0  N=10  UseFilter=on  TunerSelectOption=Transfer Function Based (PID Tuner App)  InitialConditionSource=internal  InitialConditionForIntegrator=0  InitialConditionForFilter=0  DifferentiatorICPrevScaledInput=0  ExternalReset=none  TrackingMode=off  Kt=1  LimitOutput=on  SatLimitsSource=internal  UpperSaturationLimit=2  LowerSaturationLimit=1  LinearizeAsGain=on  AntiWindupMode=clamping  Kb=1  POutMin=[]  POutMax=[]  IOutMin=[]  IOutMax=[]  DOutMin=[]  DOutMax=[]  NOutMin=[]  NOutMax=[]  SumOutMin=[]  SumOutMax=[]  SaturationOutMin=[]  SaturationOutMax=[]  PParamMin=[]  PParamMax=[]  IParamMin=[]  IParamMax=[]  DParamMin=[]  DParamMax=[]  NParamMin=[]  NParamMax=[]  KbParamMin=[]  KbParamMax=[]  KtParamMin=[]  KtParamMax=[]  KbOutMin=[]  KbOutMax=[]  KtOutMin=[]  KtOutMax=[]  IntegratorOutMin=[]  IntegratorOutMax=[]  FilterOutMin=[]  FilterOutMax=[]  SumI1OutMin=[]  SumI1OutMax=[]  SumI2OutMin=[]  SumI2OutMax=[]  SumI3OutMin=[]  SumI3OutMax=[]  SumI4OutMin=[]  SumI4OutMax=[]  SumDOutMin=[]  SumDOutMax=[]  DifferentiatorOutMin=[]  DifferentiatorOutMax=[]  FilterDiffOutCoefMin=[]  FilterDiffOutCoefMax=[]  ReciprocalOutMin=[]  ReciprocalOutMax=[]  SumDenOutMin=[]  SumDenOutMax=[]  SumNumOutMin=[]  SumNumOutMax=[]  DivideOutMin=[]  DivideOutMax=[]  UdiffTsProdOutMin=[]  UdiffTsProdOutMax=[]  NTsProdOutMin=[]  NTsProdOutMax=[]  UintegralTsProdOutMin=[]  UintegralTsProdOutMax=[]  UngainTsProdOutMin=[]  UngainTsProdOutMax=[]  IntegratorContinuousStateAttributes=''  IntegratorStateMustResolveToSignalObject=off  IntegratorRTWStateStorageClass=Auto  FilterContinuousStateAttributes=''  FilterStateMustResolveToSignalObject=off  FilterRTWStateStorageClass=Auto  ParallelPVariant=InternalParameters  IdealPVariant=Disabled  IVariant=InternalParameters  DVariant=InternalParameters  IntegratorVariant=Discrete  SatVariant=Enabled  AWVariant=DiscClampingParallel  PCopyVariant=Disabled  TRVariant=Disabled  FdbkBlocksVariant=Feedback  IdealPFdbkVariant=Passthrough  SatFdbkVariant=Passthrough  DerivativeFilterVariant=ForwardEulerFilter  NVariant=InternalParameters  NCopyVariant=Disabled  FilterICVariant=InternalICsFilter  IntegratorICVariant=InternalICs  ExternalResetVariant=Disabled  TRSumVariant=Passthrough  SumFdbkVariant=Enabled  SumVariant=Sum_PID  TsampFilterVariant=InternalTs  TsampNgainVariant=Passthrough  TsampIntegralVariant=Passthrough  ExternalSaturationOutDataTypeStr=Inherit: Same as second input  aMode=0
  Scope : Scope
  Sum{,1..3} (4 alike) : Sum  Inputs=|+-
  Unary Minus : UnaryMinus
  Unary Minus1 : UnaryMinus
  tau_Thrust : Outport
  des_pitch : Outport  Port=2
  des_roll : Outport  Port=3
  wires:
  des_alt/1 -> Sum2/1  "des_alt"
  Calculate Transformation Matrix/1(R) -> MatrixMultiply/1
  yaw_angle/1 -> Calculate Transformation Matrix/1(theta)
  Altitude Signal conditioning/1(z) -> Sum2/2  "alt"
  PID_Altitude/1 -> Sum3/1  "vz_cmd"
  vz/1 -> Unary Minus/1  "vz"
  PID_vz/1 -> Scope/1, tau_Thrust/1  "thrust_cmd"
  vx/1 -> Mux2/1  "vx"
  vy/1 -> Mux2/2  "vy"
  z/1 -> Altitude Signal conditioning/1(z_In)
  PID Controller/1 -> Demux/1
  Demux/1 -> Gain1/1
  x/1 -> Mux/1  "x"
  y/1 -> Mux/2  "y"
  Mux2/1 -> Sum/2
  Gain1/1 -> des_pitch/1
  Demux/2 -> des_roll/1
  Sum/1 -> MatrixMultiply/2
  Mux/1 -> Sum1/2
  Sum1/1 -> PID Controller1/1
  Sum3/1 -> PID_vz/1  "alt_error"
  des_x/1 -> Mux1/1  "des_x"
  des_y/1 -> Mux1/2  "des_y"
  MatrixMultiply/1 -> PID Controller/1
  PID Controller1/1 -> Sum/1
  Mux1/1 -> Sum1/1
  Sum2/1 -> Unary Minus1/1
  Unary Minus/1 -> Sum3/2
  Unary Minus1/1 -> PID_Altitude/1

== system att_control_OneModule_V6/multi Controller/Controller/Quaternion Validity Check ==
  q : Inport
  Constant : Constant  Value=[1 0 0 0]  SampleTime=-1
  Quaternion Norm : sharedutil/Quaternion Norm  aMode=aMode
      settings: SourceProductBaseCode=AE,PW,DR,MT,VE
  Switch : Switch  Criteria=u2 > Threshold  SaturateOnIntegerOverflow=off  InputSameDT=off
  Valid quat : Outport
  wires:
  q/1 -> Quaternion Norm/1, Switch/1
  Quaternion Norm/1 -> Switch/2
  Switch/1 -> Valid quat/1
  Constant/1 -> Switch/3

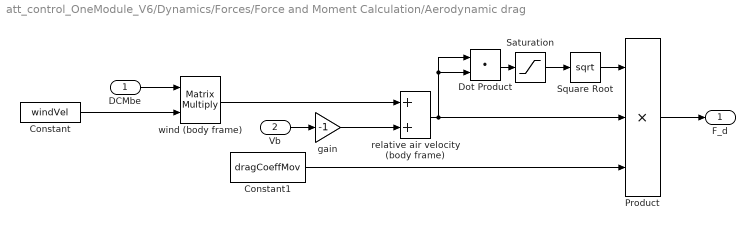
== system att_control_OneModule_V6/Dynamics/Forces/Force and Moment Calculation/Aerodynamic drag ==
  DCMbe : Inport
  Vb : Inport  Port=2
  Constant : Constant  Value=windVel
  Constant1 : Constant  Value=dragCoeffMov
  Dot Product : DotProduct  OutDataTypeStr=Inherit: Inherit via internal rule
  Product : Product  Inputs=3
  Saturation : Saturate  UpperLimit=inf  LowerLimit=0.0001
  Square Root : Sqrt
  gain : Gain  Gain=-1
  relative air velocity (body frame) : Sum
  wind (body frame) : Product  Multiplication=Matrix(*)
  F_d : Outport
  wires:
  relative air velocity (body frame)/1 -> Dot Product/2, Dot Product/1, Product/2
  DCMbe/1 -> wind (body frame)/1
  Product/1 -> F_d/1
  Saturation/1 -> Square Root/1
  Vb/1 -> gain/1
  Dot Product/1 -> Saturation/1
  Square Root/1 -> Product/1
  wind (body frame)/1 -> relative air velocity (body frame)/1
  gain/1 -> relative air velocity (body frame)/2
  Constant1/1 -> Product/3
  Constant/1 -> wind (body frame)/2

== system att_control_OneModule_V6/Dynamics/Forces/Force and Moment Calculation/Gravity ==
  DCM_be : Inport
  Constant : Constant  Value=[0 0 g]'
  Gain : Gain  Gain=mass
  Matrix Multiply : Product  Multiplication=Matrix(*)
  F_g : Outport
  wires:
  Matrix Multiply/1 -> Gain/1
  Constant/1 -> Matrix Multiply/2
  DCM_be/1 -> Matrix Multiply/1
  Gain/1 -> F_g/1

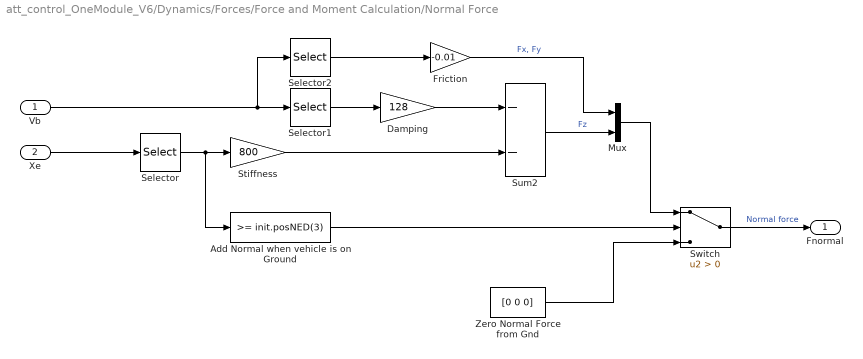
== system att_control_OneModule_V6/Dynamics/Forces/Force and Moment Calculation/Normal Force ==
  Vb : Inport
  Xe : Inport  Port=2
  Add Normal when vehicle is on Ground : simulink/Logic and Bit Operations/Compare To Constant  relop=>=  const=init.posNED(3)  OutDataTypeStr=boolean
  Damping : Gain  Gain=128  SaturateOnIntegerOverflow=on  OutDataTypeStr=Inherit: Same as input  ParamDataTypeStr=Inherit: Same as input
  Friction : Gain  Gain=-0.01
  Mux : Mux  Inputs=2
  Selector : Selector  InputPortWidth=3  IndexOptions=Index vector (dialog)  Indices=[3]  OutputSizes=1
  Selector1 : Selector  InputPortWidth=3  IndexOptions=Index vector (dialog)  Indices=[3]  OutputSizes=1
  Selector2 : Selector  InputPortWidth=3  IndexOptions=Index vector (dialog)  Indices=[1 2]  OutputSizes=1
  Stiffness : Gain  Gain=800  SaturateOnIntegerOverflow=on  OutDataTypeStr=Inherit: Same as input  ParamDataTypeStr=Inherit: Same as input
  Sum2 : Sum  Inputs=--  InputSameDT=on  SaturateOnIntegerOverflow=on  OutDataTypeStr=Inherit: Same as first input
  Switch : Switch  Criteria=u2 > Threshold  SaturateOnIntegerOverflow=off  InputSameDT=off
  Zero Normal Force from Gnd : Constant  Value=[0 0 0]  SampleTime=-1
  Fnormal : Outport
  wires:
  Selector/1 -> Stiffness/1, Add Normal when vehicle is on Ground/1
  Stiffness/1 -> Sum2/2
  Damping/1 -> Sum2/1
  Sum2/1 -> Mux/2  "Fz"
  Xe/1 -> Selector/1
  Add Normal when vehicle is on Ground/1 -> Switch/2
  Selector1/1 -> Damping/1
  Vb/1 -> Selector2/1, Selector1/1
  Zero Normal Force from Gnd/1 -> Switch/3
  Friction/1 -> Mux/1  "Fx, Fy"
  Selector2/1 -> Friction/1
  Mux/1 -> Switch/1
  Switch/1 -> Fnormal/1  "Normal force"
